simulink model "Simulation_straight_line"  (R2017b)
settings: Solver=ode45  StartTime=0.0  StopTime=inf  RelTol=1e-3  EnableMultiTasking=on
values from neighbouring files (symbols this model uses):
  s = zc-d1    [ArticuledManipulator_Ik.m]
undefined symbols (not defined in the file or in its folder): baza, efector, flansa, robot_nou, RootGround, RootPart, rv
libraries: mblibv1 x31, vrlib x8, simulink x1
settings Model: Creator=elod  LastModifiedBy=Rodrigo Chi
settings DataIOCC: LimitDataPoints=on  SaveFormat=Array  SignalLoggingSaveFormat=ModelDataLogs
settings OptimizationCC: ExpressionDepthLimit=2147483647  LifeSpan=inf
settings DebuggingCC: AlgebraicLoopMsg=none  UnderspecifiedInitializationDetection=Classic  MergeDetectMultiDrivingBlocksExec=none  SolverPrmCheckMsg=warning  FcnCallInpInsideContextMsg=warning  StateNameClashWarn=warning  SFUnexpectedBacktrackingDiag=warning  SFNoUnconditionalDefaultTransitionDiag=warning  SFExecutionAtInitializationDiag=none
settings HardwareCC: ProdBitPerPointer=32  ProdBitPerSizeT=32  ProdBitPerPtrDiffT=32  ProdLargestAtomicFloat=None  ProdIntDivRoundTo=Undefined  ProdEndianess=Unspecified  ProdWordSize=32  ProdHWDeviceType=32-bit Generic
settings ModelReferenceCC: PropagateSignalLabelsOutOfModel=off
settings CodeAppCC: StateflowObjectComments=on
settings GRTTargetCC: TargetLangStandard=C89/C90 (ANSI)  GeneratePreprocessorConditionals=Disable all  CombineOutputUpdateFcns=off  GRTInterface=on
settings ConfigComp: CovMetricSettings=dw  CovHtmlReporting=on  CovSaveCumulativeToWorkspaceVar=on  CovSaveSingleToWorkspaceVar=on  CovExternalEMLEnable=off
settings SimscapeCC: SimscapeNormalizeSystem=off
settings SimMechanicsCC: VisOnUpdateDiagram=on  VisDuringSimulation=on

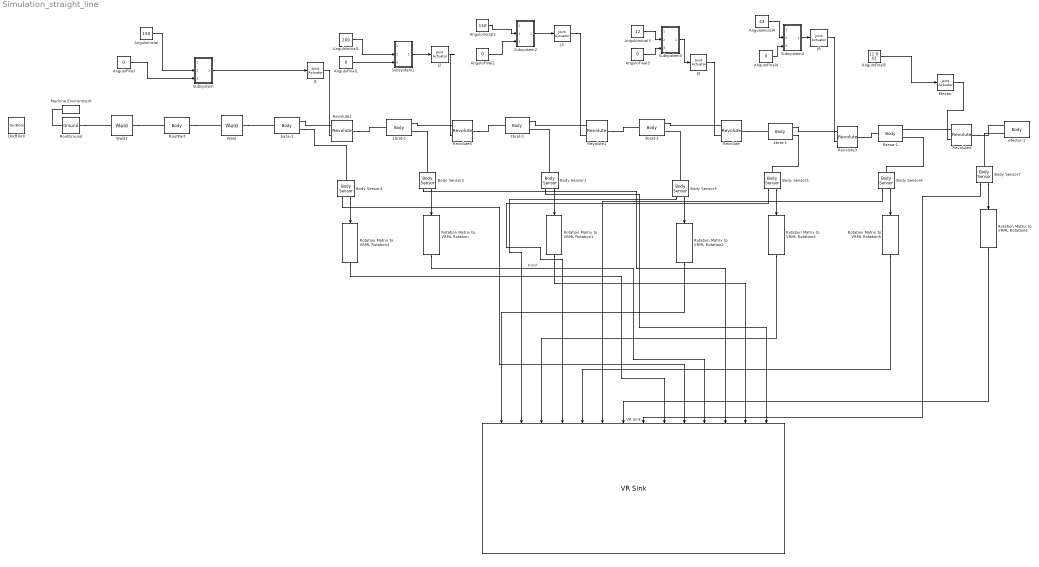
== system Simulation_straight_line ==
  1brat-1 : mblibv1/Bodies/Body  LConnTagsString=CS2  RConnTagsString=CS3|CS4  UpdateFromCAD=on  PMImportedID=1brat-1  DialogClass=MechanicalBodyBlock  Mass=2.25015  MassUnits=kg  InertiaUnits=kg*m^2  Inertia=[0.00885227,-5.51348e-008,-0.000219712;-5.51348e-008,0.00930047,6.21532e-009;-0.000219712,6.21532e-009,0.00500541]  Shape=Cylinder  ShapeDims=[1 1]  ShapeUnits=m  ShapeUse=false  Density=1  DensityUnits=kg/m^3  DensityUse=false  GraphicsMode=GFXFILE  GraphicsFileName=C:\Users\Rodrigo Chi\Desktop\Robot_Melfa\robot_nou - 1brat-1.STL  BodyColorSelMode=COLORPALETTE  BodyColor=[0.65098;0.65098;0.65098]  AttachedToCS=CS1  CG=Right$CG$[0.00726331 0.0794388 -8.78869e-008]$WORLD$WORLD$m$[-1 0 0;0 0 1;0 1 0]$3x3 Transform$rad$WORLD$false$1brat-1::CG(AUTOGEN)  WorkingFrames=Right$CS1$[0 -0.00299998 0]$WORLD$WORLD$m$[-1 0 0;0 0 1;0 1 0]$3x3 Transform$rad$WORLD$false$1brat-1::CS1(AUTOGEN)#Left$CS2$[-1.38778e-017 2.5e-008 5.8564e-016]$WORLD$WORLD$m$[1 0 0;0 1 0;0 0 1]$3x3 Transform$rad$WORLD$true$1brat-1:-:baza-1::1brat-1(AUTOGEN)#Right$CS3$[0 0.1295 -0.0448145]$WORLD$WORLD$m$[1 0 0;0 1 0;0 0 1]$3x3 Transform$rad$WORLD$true$1brat-1:-:2brat-1::1brat-1(AUTOGEN)#Right$CS4$[0 0 0]$WORLD$WORLD$m$[1 0 0;0 1 0;0 0 1]$3x3 Transform$rad$WORLD$true$none  CGPos=[0.00726331 0.0794388 -8.78869e-008]  CGRot=[-1 0 0;0 0 1;0 1 0]  CS0Pos=[]  CS0Rot=[]  CS1Pos=[0 -0.00299998 0]  CS1Rot=[-1 0 0;0 0 1;0 1 0]  CS2Pos=[-1.38778e-017 2.5e-008 5.8564e-016]  CS2Rot=[1 0 0;0 1 0;0 0 1]  CS3Pos=[0 0.1295 -0.0448145]  CS3Rot=[1 0 0;0 1 0;0 0 1]  CS4Pos=[0 0 0]  CS4Rot=[1 0 0;0 1 0;0 0 1]  CS5Pos=[]  CS5Rot=[]  CS6Pos=[]  CS6Rot=[]  CS7Pos=[]  CS7Rot=[]  CS8Pos=[]  CS8Rot=[]  CS9Pos=[]  CS9Rot=[]  CS10Pos=[]  CS10Rot=[]  CS11Pos=[]  CS11Rot=[]  CS12Pos=[]  CS12Rot=[]  CS13Pos=[]  CS13Rot=[]  CS14Pos=[]  CS14Rot=[]  CS15Pos=[]  CS15Rot=[]  CS16Pos=[]  CS16Rot=[]  CS17Pos=[]  CS17Rot=[]  CS18Pos=[]  CS18Rot=[]  CS19Pos=[]  CS19Rot=[]  CS20Pos=[]  CS20Rot=[]
      settings: SourceProductName=Simscape Multibody  SourceProductBaseCode=MS
  2brat-1 : mblibv1/Bodies/Body  LConnTagsString=CS3  RConnTagsString=CS2|CS4  UpdateFromCAD=on  PMImportedID=2brat-1  DialogClass=MechanicalBodyBlock  Mass=3.62743  MassUnits=kg  InertiaUnits=kg*m^2  Inertia=[0.0393757,-7.68618e-009,0.000126615;-7.68618e-009,0.0293486,-4.48119e-008;0.000126615,-4.48119e-008,0.0153003]  Shape=Cylinder  ShapeDims=[1 1]  ShapeUnits=m  ShapeUse=false  Density=1  DensityUnits=kg/m^3  DensityUse=false  GraphicsMode=GFXFILE  GraphicsFileName=C:\Users\Rodrigo Chi\Desktop\Robot_Melfa\robot_nou - 2brat-1.STL  BodyColorSelMode=COLORPALETTE  BodyColor=[0.65098;0.65098;0.65098]  AttachedToCS=CS1  CG=Right$CG$[-0.000659844 0.24353 1.10558e-006]$WORLD$WORLD$m$[1 0 0;0 0 1;0 -1 0]$3x3 Transform$rad$WORLD$false$2brat-1::CG(AUTOGEN)  WorkingFrames=Right$CS1$[0 0.1295 0]$WORLD$WORLD$m$[1 0 0;0 0 1;0 -1 0]$3x3 Transform$rad$WORLD$false$2brat-1::CS1(AUTOGEN)#Right$CS2$[0 0.3795 0.0880007]$WORLD$WORLD$m$[1 0 0;0 1 0;0 0 1]$3x3 Transform$rad$WORLD$true$2brat-1:-:3brat-1::2brat-1(AUTOGEN)#Left$CS3$[0 0.1295 -0.0448145]$WORLD$WORLD$m$[1 0 0;0 1 0;0 0 1]$3x3 Transform$rad$WORLD$true$1brat-1:-:2brat-1::2brat-1(AUTOGEN)#Right$CS4$[0 0 0]$WORLD$WORLD$m$[1 0 0;0 1 0;0 0 1]$3x3 Transform$rad$WORLD$true$none  CGPos=[-0.000659844 0.24353 1.10558e-006]  CGRot=[1 0 0;0 0 1;0 -1 0]  CS0Pos=[]  CS0Rot=[]  CS1Pos=[0 0.1295 0]  CS1Rot=[1 0 0;0 0 1;0 -1 0]  CS2Pos=[0 0.3795 0.0880007]  CS2Rot=[1 0 0;0 1 0;0 0 1]  CS3Pos=[0 0.1295 -0.0448145]  CS3Rot=[1 0 0;0 1 0;0 0 1]  CS4Pos=[0 0 0]  CS4Rot=[1 0 0;0 1 0;0 0 1]  CS5Pos=[]  CS5Rot=[]  CS6Pos=[]  CS6Rot=[]  CS7Pos=[]  CS7Rot=[]  CS8Pos=[]  CS8Rot=[]  CS9Pos=[]  CS9Rot=[]  CS10Pos=[]  CS10Rot=[]  CS11Pos=[]  CS11Rot=[]  CS12Pos=[]  CS12Rot=[]  CS13Pos=[]  CS13Rot=[]  CS14Pos=[]  CS14Rot=[]  CS15Pos=[]  CS15Rot=[]  CS16Pos=[]  CS16Rot=[]  CS17Pos=[]  CS17Rot=[]  CS18Pos=[]  CS18Rot=[]  CS19Pos=[]  CS19Rot=[]  CS20Pos=[]  CS20Rot=[]
      settings: SourceProductName=Simscape Multibody  SourceProductBaseCode=MS
  3brat-1 : mblibv1/Bodies/Body  LConnTagsString=CS3  RConnTagsString=CS2|CS4  UpdateFromCAD=on  PMImportedID=3brat-1  DialogClass=MechanicalBodyBlock  Mass=1.71089  MassUnits=kg  InertiaUnits=kg*m^2  Inertia=[0.00842552,-6.36697e-007,1.27806e-006;-6.36697e-007,0.00773782,1.23963e-005;1.27806e-006,1.23963e-005,0.00280267]  Shape=Cylinder  ShapeDims=[1 1]  ShapeUnits=m  ShapeUse=false  Density=1  DensityUnits=kg/m^3  DensityUse=false  GraphicsMode=GFXFILE  GraphicsFileName=C:\Users\Rodrigo Chi\Desktop\Robot_Melfa\robot_nou - 3brat-1.STL  BodyColorSelMode=COLORPALETTE  BodyColor=[0.65098;0.65098;0.65098]  AttachedToCS=CS1  CG=Right$CG$[7.52531e-006 0.448063 0.00032452]$WORLD$WORLD$m$[1 0 0;0 0 1;0 -1 0]$3x3 Transform$rad$WORLD$false$3brat-1::CG(AUTOGEN)  WorkingFrames=Right$CS1$[0 0.3795 0]$WORLD$WORLD$m$[1 0 0;0 0 1;0 -1 0]$3x3 Transform$rad$WORLD$false$3brat-1::CS1(AUTOGEN)#Right$CS2$[-0.000180127 0.5395 -0.0224506]$WORLD$WORLD$m$[1 0 0;0 1 0;0 0 1]$3x3 Transform$rad$WORLD$true$3brat-1:-:4brat-1::3brat-1(AUTOGEN)#Left$CS3$[0 0.3795 0.0880007]$WORLD$WORLD$m$[1 0 0;0 1 0;0 0 1]$3x3 Transform$rad$WORLD$true$2brat-1:-:3brat-1::3brat-1(AUTOGEN)#Right$CS4$[0 0 0]$WORLD$WORLD$m$[1 0 0;0 1 0;0 0 1]$3x3 Transform$rad$WORLD$true$none  CGPos=[7.52531e-006 0.448063 0.00032452]  CGRot=[1 0 0;0 0 1;0 -1 0]  CS0Pos=[]  CS0Rot=[]  CS1Pos=[0 0.3795 0]  CS1Rot=[1 0 0;0 0 1;0 -1 0]  CS2Pos=[-0.000180127 0.5395 -0.0224506]  CS2Rot=[1 0 0;0 1 0;0 0 1]  CS3Pos=[0 0.3795 0.0880007]  CS3Rot=[1 0 0;0 1 0;0 0 1]  CS4Pos=[0 0 0]  CS4Rot=[1 0 0;0 1 0;0 0 1]  CS5Pos=[]  CS5Rot=[]  CS6Pos=[]  CS6Rot=[]  CS7Pos=[]  CS7Rot=[]  CS8Pos=[]  CS8Rot=[]  CS9Pos=[]  CS9Rot=[]  CS10Pos=[]  CS10Rot=[]  CS11Pos=[]  CS11Rot=[]  CS12Pos=[]  CS12Rot=[]  CS13Pos=[]  CS13Rot=[]  CS14Pos=[]  CS14Rot=[]  CS15Pos=[]  CS15Rot=[]  CS16Pos=[]  CS16Rot=[]  CS17Pos=[]  CS17Rot=[]  CS18Pos=[]  CS18Rot=[]  CS19Pos=[]  CS19Rot=[]  CS20Pos=[]  CS20Rot=[]
      settings: SourceProductName=Simscape Multibody  SourceProductBaseCode=MS
  4brat-1 : mblibv1/Bodies/Body  LConnTagsString=CS2  RConnTagsString=CS3|CS4  UpdateFromCAD=on  PMImportedID=4brat-1  DialogClass=MechanicalBodyBlock  Mass=0.330921  MassUnits=kg  InertiaUnits=kg*m^2  Inertia=[0.000305863,9.08861e-011,-3.82551e-010;9.08861e-011,0.000416962,-1.09526e-009;-3.82551e-010,-1.09526e-009,0.000217954]  Shape=Cylinder  ShapeDims=[1 1]  ShapeUnits=m  ShapeUse=false  Density=1  DensityUnits=kg/m^3  DensityUse=false  GraphicsMode=GFXFILE  GraphicsFileName=C:\Users\Rodrigo Chi\Desktop\Robot_Melfa\robot_nou - 4brat-1.STL  BodyColorSelMode=COLORPALETTE  BodyColor=[0.65098;0.65098;0.65098]  AttachedToCS=CS1  CG=Right$CG$[-0.000180145 0.534322 2.80673e-008]$WORLD$WORLD$m$[1 0 0;0 0 1;0 -1 0]$3x3 Transform$rad$WORLD$false$4brat-1::CG(AUTOGEN)  WorkingFrames=Right$CS1$[-0.000180127 0.5395 0]$WORLD$WORLD$m$[1 0 0;0 0 1;0 -1 0]$3x3 Transform$rad$WORLD$false$4brat-1::CS1(AUTOGEN)#Left$CS2$[-0.000180127 0.5395 -0.0224506]$WORLD$WORLD$m$[1 0 0;0 1 0;0 0 1]$3x3 Transform$rad$WORLD$true$3brat-1:-:4brat-1::4brat-1(AUTOGEN)#Right$CS3$[-0.000180127 0.5855 0]$WORLD$WORLD$m$[1 0 0;0 1 0;0 0 1]$3x3 Transform$rad$WORLD$true$4brat-1:-:flansa-1::4brat-1(AUTOGEN)#Right$CS4$[0 0 0]$WORLD$WORLD$m$[1 0 0;0 1 0;0 0 1]$3x3 Transform$rad$WORLD$true$none  CGPos=[-0.000180145 0.534322 2.80673e-008]  CGRot=[1 0 0;0 0 1;0 -1 0]  CS0Pos=[]  CS0Rot=[]  CS1Pos=[-0.000180127 0.5395 0]  CS1Rot=[1 0 0;0 0 1;0 -1 0]  CS2Pos=[-0.000180127 0.5395 -0.0224506]  CS2Rot=[1 0 0;0 1 0;0 0 1]  CS3Pos=[-0.000180127 0.5855 0]  CS3Rot=[1 0 0;0 1 0;0 0 1]  CS4Pos=[0 0 0]  CS4Rot=[1 0 0;0 1 0;0 0 1]  CS5Pos=[]  CS5Rot=[]  CS6Pos=[]  CS6Rot=[]  CS7Pos=[]  CS7Rot=[]  CS8Pos=[]  CS8Rot=[]  CS9Pos=[]  CS9Rot=[]  CS10Pos=[]  CS10Rot=[]  CS11Pos=[]  CS11Rot=[]  CS12Pos=[]  CS12Rot=[]  CS13Pos=[]  CS13Rot=[]  CS14Pos=[]  CS14Rot=[]  CS15Pos=[]  CS15Rot=[]  CS16Pos=[]  CS16Rot=[]  CS17Pos=[]  CS17Rot=[]  CS18Pos=[]  CS18Rot=[]  CS19Pos=[]  CS19Rot=[]  CS20Pos=[]  CS20Rot=[]
      settings: SourceProductName=Simscape Multibody  SourceProductBaseCode=MS
  AnguloFinal{,1..4} (5 alike) : Constant  Value=0
  AnguloFinal5 : Constant  Value=[1 0 0]
  AnguloInicial : Constant  Value=150
  AnguloInicial1 : Constant  Value=200
  AnguloInicial2 : Constant  Value=150
  AnguloInicial3 : Constant  Value=12
  AnguloInicial4 : Constant  Value=44
  Body Sensor{1..7} (7 alike) : mblibv1/Sensors &  Actuators/Body Sensor  UpdateFromCAD=off  PhysicalDomain=Mechanical  PortType=blob  Muxed=off  Pose=on  Angle=on  AngleUnits=deg  ArcVelocity=off  ArcVelocityUnits=deg/s  ArcAcceleration=off  ArcAccelerationUnits=deg/s^2  CoordPosition=on  CoordPositionUnits=m  Velocity=off  VelocityUnits=m/s  Acceleration=off  AccelerationUnits=m/s^2  Quaternion=on  QuaternionDT=off  QuaternionDDT=off  QuaternionUnits=off  OutputVector=[1]  ActiveIO=on  Width=12  DialogClass=MechanicalSensorBlock  ReferenceFrame=Absolute (World)
      settings: SourceProductName=Simscape Multibody  SourceProductBaseCode=MS
  DocBlock : simulink/Model-Wide Utilities/DocBlock  DocumentType=Text
      content=|
      | Type your documentation here
      | el robot funcioa por bloques y los ejes de rotacion estan unidos
      | a actuadores que a su vez reciben 3 constantes ed las cuales
      | 1 se puede cambiar usando el slider
      |
      | cada eje(revolute) esta basado en l eje del robot
      | hay algunos que solo giran en x y otros en y etc
      | para la manipulacion se usa el slider gain con un rango de -180
      | a 180
      |
      | los join actuator se deben cambiar de "generalized forces" a
      | "motion" para poder ser manipulados
  Efector : mblibv1/Sensors &  Actuators/Joint Actuator  UpdateFromCAD=off  PhysicalDomain=Mechanical  PortType=blob  ActuationStyle=Motion  AngleUnits=deg  ArcVelocityUnits=deg/s  ArcAccelerationUnits=deg/s^2  CoordPositionUnits=m  VelocityUnits=m/s  AccelerationUnits=m/s^2  ForceUnits=N  TorqueUnits=N*m  ActiveIO=on  Width=3  DialogClass=MechanicalActuatorBlock  Primitive=R1  ReferenceFrame=Absolute (World)
      settings: SourceProductName=Simscape Multibody  SourceProductBaseCode=MS
  J{1..3,5..6} (5 alike) : mblibv1/Sensors &  Actuators/Joint Actuator  UpdateFromCAD=off  PhysicalDomain=Mechanical  PortType=blob  ActuationStyle=Motion  AngleUnits=deg  ArcVelocityUnits=deg/s  ArcAccelerationUnits=deg/s^2  CoordPositionUnits=m  VelocityUnits=m/s  AccelerationUnits=m/s^2  ForceUnits=N  TorqueUnits=N*m  ActiveIO=on  Width=3  DialogClass=MechanicalActuatorBlock  Primitive=R1  ReferenceFrame=Absolute (World)
      settings: SourceProductName=Simscape Multibody  SourceProductBaseCode=MS
  Machine Environment : mblibv1/Bodies/Machine Environment  PortType=env  PhysicalDomain=Mechanical  DialogTemplateClass=MECH.MachineEnvironment  SyncWhenCopied=off  Gravity=[0 -9.81 0]  GravityUnits=m/s^2  GravityAsSignal=off  Dimensionality=Auto-detect  AnalysisType=Forward dynamics  LinearAssemblyTolerance=1e-3  LinearAssemblyToleranceUnits=m  AngularAssemblyTolerance=1e-3  AngularAssemblyToleranceUnits=rad  ConstraintSolverType=Stabilizing  ConstraintRelTolerance=1e-4  ConstraintAbsTolerance=1e-4  UseRobustSingularityHandling=off  RedundancyAnalysisToleranceType=Automatically select tolerance  RedundancyAnalysisTolerance=1e-14  StatePerturbationType=Fixed  PerturbationSize=1e-5  VisualizeMachine=on  BodyVisualizationType=Use model default body geometries  BodyColorSelMode=Use model default  DefaultBodyColor=[1 0 0]
      settings: SourceProductName=Simscape Multibody  SourceProductBaseCode=MS
  Revolute : mblibv1/Joints/Revolute  LConnTagsString=__newl0|SA1  RConnTagsString=__newr0  UpdateFromCAD=on  PMImportedID=3brat-1:-:4brat-1  NumSAPorts=1  CutJoint=off  MarkAsCut=off  Primitives=prismatic  PrimitiveProps=R1$World$[0,0,-1]$revolute  DialogClass=JointBlock  R1Axis=[0,0,-1]
      settings: SourceProductName=Simscape Multibody  SourceProductBaseCode=MS
  Revolute1 : mblibv1/Joints/Revolute  LConnTagsString=__newl0|SA1  RConnTagsString=__newr0  UpdateFromCAD=on  PMImportedID=2brat-1:-:3brat-1  NumSAPorts=1  CutJoint=off  MarkAsCut=off  Primitives=prismatic  PrimitiveProps=R1$World$[0,0,-1]$revolute  DialogClass=JointBlock  R1Axis=[0,0,-1]
      settings: SourceProductName=Simscape Multibody  SourceProductBaseCode=MS
  Revolute2 : mblibv1/Joints/Revolute  LConnTagsString=__newl0|SA1  RConnTagsString=__newr0  UpdateFromCAD=on  PMImportedID=1brat-1:-:baza-1  NumSAPorts=1  CutJoint=off  MarkAsCut=off  Primitives=prismatic  PrimitiveProps=R1$World$[0,1,0]$revolute  DialogClass=JointBlock  R1Axis=[0,1,0]
      settings: SourceProductName=Simscape Multibody  SourceProductBaseCode=MS
  Revolute3 : mblibv1/Joints/Revolute  LConnTagsString=__newl0|SA1  RConnTagsString=__newr0  UpdateFromCAD=on  PMImportedID=4brat-1:-:flansa-1  NumSAPorts=1  CutJoint=off  MarkAsCut=off  Primitives=prismatic  PrimitiveProps=R1$World$[0,1,0]$revolute  DialogClass=JointBlock  R1Axis=[0,1,0]
      settings: SourceProductName=Simscape Multibody  SourceProductBaseCode=MS
  Revolute4 : mblibv1/Joints/Revolute  LConnTagsString=__newl0|SA1  RConnTagsString=__newr0  UpdateFromCAD=on  PMImportedID=efector-1:-:flansa-1  NumSAPorts=1  CutJoint=off  MarkAsCut=off  Primitives=prismatic  PrimitiveProps=R1$World$[0,1,0]$revolute  DialogClass=JointBlock  R1Axis=[0,1,0]
      settings: SourceProductName=Simscape Multibody  SourceProductBaseCode=MS
  Revolute5 : mblibv1/Joints/Revolute  LConnTagsString=__newl0|SA1  RConnTagsString=__newr0  UpdateFromCAD=on  PMImportedID=1brat-1:-:2brat-1  NumSAPorts=1  CutJoint=off  MarkAsCut=off  Primitives=prismatic  PrimitiveProps=R1$World$[0,0,1]$revolute  DialogClass=JointBlock  R1Axis=[0,0,1]
      settings: SourceProductName=Simscape Multibody  SourceProductBaseCode=MS
  RootGround : mblibv1/Bodies/Ground  UpdateFromCAD=on  PMImportedID=RootGround  LeftPortType=env  RightPortType=workingframe  PhysicalDomain=Mechanical  DialogClass=GroundBlock  CoordPosition=[0.0162361,0.125438,4.43298e-005]  CoordPositionUnits=m  StateVectorMgrId=3  MachineId=[4 0]  ShowEnvPort=on  ParameterChecksum=[727912128, 70383034, 523039224, 3416024631]  TopologyChecksum=[549250593, 3930916714, 1254666677, 4177042960]
      settings: SourceProductName=Simscape Multibody  SourceProductBaseCode=MS
  RootPart : mblibv1/Bodies/Body  LConnTagsString=CS3  RConnTagsString=CS2  UpdateFromCAD=on  PMImportedID=robot_nou/RootPart  DialogClass=MechanicalBodyBlock  Mass=0  MassUnits=kg  InertiaUnits=kg*m^2  Inertia=[0,0,0;0,0,0;0,0,0]  Shape=Cylinder  ShapeDims=[1 1]  ShapeUnits=m  ShapeUse=false  Density=1  DensityUnits=kg/m^3  DensityUse=false  GraphicsMode=GFXFILE  GraphicsFileName=C:\Users\Rodrigo Chi\Desktop\Robot Físico Geo\Robotsimulado\robot_nou - baza-1.STL  BodyColorSelMode=COLORPALETTE  BodyColor=[0.501961;0.501961;0.501961]  AttachedToCS=CS1  CG=Right$CG$[0.0162361 0.125438 4.43298e-005]$WORLD$WORLD$m$[1 0 0;0 1 0;0 0 1]$3x3 Transform$rad$WORLD$false$robot_nou/RootPart::CG(AUTOGEN)  WorkingFrames=Right$CS1$[0 0 0]$WORLD$WORLD$m$[1 0 0;0 1 0;0 0 1]$3x3 Transform$rad$WORLD$false$robot_nou/RootPart::CS1(AUTOGEN)#Right$CS2$[0.0387863 -0.0914613 7.26852e-006]$WORLD$WORLD$m$[1 0 0;0 1 0;0 0 1]$3x3 Transform$rad$WORLD$true$baza-1:-:robot_nou/RootPart::robot_nou/RootPart(AUTOGEN)#Left$CS3$[0.0162361 0.125438 4.43298e-005]$WORLD$WORLD$m$[1 0 0;0 1 0;0 0 1]$3x3 Transform$rad$WORLD$true$RootGround:-:robot_nou/RootPart::robot_nou/RootPart(AUTOGEN)  CGPos=[0.0162361 0.125438 4.43298e-005]  CGRot=[1 0 0;0 1 0;0 0 1]  CS0Pos=[]  CS0Rot=[]  CS1Pos=[0 0 0]  CS1Rot=[1 0 0;0 1 0;0 0 1]  CS2Pos=[0.0387863 -0.0914613 7.26852e-006]  CS2Rot=[1 0 0;0 1 0;0 0 1]  CS3Pos=[0.0162361 0.125438 4.43298e-005]  CS3Rot=[1 0 0;0 1 0;0 0 1]  CS4Pos=[]  CS4Rot=[]  CS5Pos=[]  CS5Rot=[]  CS6Pos=[]  CS6Rot=[]  CS7Pos=[]  CS7Rot=[]  CS8Pos=[]  CS8Rot=[]  CS9Pos=[]  CS9Rot=[]  CS10Pos=[]  CS10Rot=[]  CS11Pos=[]  CS11Rot=[]  CS12Pos=[]  CS12Rot=[]  CS13Pos=[]  CS13Rot=[]  CS14Pos=[]  CS14Rot=[]  CS15Pos=[]  CS15Rot=[]  CS16Pos=[]  CS16Rot=[]  CS17Pos=[]  CS17Rot=[]  CS18Pos=[]  CS18Rot=[]  CS19Pos=[]  CS19Rot=[]  CS20Pos=[]  CS20Rot=[]
      settings: SourceProductName=Simscape Multibody  SourceProductBaseCode=MS
  Rotation Matrix to VRML Rotation{,1..6} (7 alike) : vrlib/Utilities/Rotation Matrix to VRML Rotation  maxzero=1e-12
      settings: SourceProductName=Simulink 3D Animation  SourceProductBaseCode=VR
  Subsystem : Subsystem
  Subsystem1 : Subsystem
  Subsystem2 : Subsystem
  Subsystem3 : Subsystem
  Subsystem4 : Subsystem
  VR Sink : vrlib/VR Sink  InstantiateOnLoad=on  SampleTime=0.1  ViewEnable=on  RemoteChange=off  RemoteView=off  FieldsWritten=b3.rotation.4.1.1.double#b3.translation.3.1.1.double#b4.rotation.4.1.1.double#b4.translation.3.1.1.double#f.rotation.4.1.1.double#f.translation.3.1.1.double#e.rotation.4.1.1.double#e.translation.3.1.1.double#bb.rotation.4.1.1.double#bb.translation.3.1.1.double#b1.rotation.4.1.1.double#b1.translation.3.1.1.double#b2.rotation.4.1.1.double#b2.translation.3.1.1.double  WorldFileName=robot_Rva2j.wrl  WorldDescription=rv-2aj  AutoView=off  VideoDimensions=[]  AllowVariableSize=off
      settings: SourceProductBaseCode=VR
  Weld : mblibv1/Joints/Weld  LConnTagsString=__newl0  RConnTagsString=__newr0  UpdateFromCAD=on  PMImportedID=baza-1:-:robot_nou/RootPart  NumSAPorts=0  CutJoint=off  MarkAsCut=off  Primitives=weld  PrimitiveProps=W$WORLD$[0.57735,0.57735,0.57735]$weld  DialogClass=JointBlock  WAxis=[0.57735,0.57735,0.57735]
      settings: SourceProductName=Simscape Multibody  SourceProductBaseCode=MS
  Weld1 : mblibv1/Joints/Weld  LConnTagsString=__newl0  RConnTagsString=__newr0  UpdateFromCAD=on  PMImportedID=RootGround:-:robot_nou/RootPart  NumSAPorts=0  CutJoint=off  MarkAsCut=off  Primitives=weld  PrimitiveProps=W$WORLD$[0.57735,0.57735,0.57735]$weld  DialogClass=JointBlock  WAxis=[0.57735,0.57735,0.57735]
      settings: SourceProductName=Simscape Multibody  SourceProductBaseCode=MS
  baza-1 : mblibv1/Bodies/Body  LConnTagsString=CS2  RConnTagsString=CS3|CS4  UpdateFromCAD=on  PMImportedID=baza-1  DialogClass=MechanicalBodyBlock  Mass=5.28442  MassUnits=kg  InertiaUnits=kg*m^2  Inertia=[0.0219514,4.64467e-006,-0.00187329;4.64467e-006,0.0327268,7.62797e-007;-0.00187329,7.62797e-007,0.0305246]  Shape=Cylinder  ShapeDims=[1 1]  ShapeUnits=m  ShapeUse=false  Density=1  DensityUnits=kg/m^3  DensityUse=false  GraphicsMode=GFXFILE  GraphicsFileName=C:\Users\Rodrigo Chi\Desktop\Robot_Melfa\robot_nou - baza-1.STL  BodyColorSelMode=COLORPALETTE  BodyColor=[0.65098;0.65098;0.65098]  AttachedToCS=CS1  CG=Right$CG$[0.0387863 -0.0914613 7.26852e-006]$WORLD$WORLD$m$[-1 0 0;0 0 1;0 1 0]$3x3 Transform$rad$WORLD$false$baza-1::CG(AUTOGEN)  WorkingFrames=Right$CS1$[0 -0.168 0]$WORLD$WORLD$m$[-1 0 0;0 0 1;0 1 0]$3x3 Transform$rad$WORLD$false$baza-1::CS1(AUTOGEN)#Left$CS2$[0.0387863 -0.0914613 7.26852e-006]$WORLD$WORLD$m$[1 0 0;0 1 0;0 0 1]$3x3 Transform$rad$WORLD$true$baza-1:-:robot_nou/RootPart::baza-1(AUTOGEN)#Right$CS3$[-1.38778e-017 2.5e-008 5.8564e-016]$WORLD$WORLD$m$[1 0 0;0 1 0;0 0 1]$3x3 Transform$rad$WORLD$true$1brat-1:-:baza-1::baza-1(AUTOGEN)#Right$CS4$[0 0 0]$WORLD$WORLD$m$[1 0 0;0 1 0;0 0 1]$3x3 Transform$rad$WORLD$true$none  CGPos=[0.0387863 -0.0914613 7.26852e-006]  CGRot=[-1 0 0;0 0 1;0 1 0]  CS0Pos=[]  CS0Rot=[]  CS1Pos=[0 -0.168 0]  CS1Rot=[-1 0 0;0 0 1;0 1 0]  CS2Pos=[0.0387863 -0.0914613 7.26852e-006]  CS2Rot=[1 0 0;0 1 0;0 0 1]  CS3Pos=[-1.38778e-017 2.5e-008 5.8564e-016]  CS3Rot=[1 0 0;0 1 0;0 0 1]  CS4Pos=[0 0 0]  CS4Rot=[1 0 0;0 1 0;0 0 1]  CS5Pos=[]  CS5Rot=[]  CS6Pos=[]  CS6Rot=[]  CS7Pos=[]  CS7Rot=[]  CS8Pos=[]  CS8Rot=[]  CS9Pos=[]  CS9Rot=[]  CS10Pos=[]  CS10Rot=[]  CS11Pos=[]  CS11Rot=[]  CS12Pos=[]  CS12Rot=[]  CS13Pos=[]  CS13Rot=[]  CS14Pos=[]  CS14Rot=[]  CS15Pos=[]  CS15Rot=[]  CS16Pos=[]  CS16Rot=[]  CS17Pos=[]  CS17Rot=[]  CS18Pos=[]  CS18Rot=[]  CS19Pos=[]  CS19Rot=[]  CS20Pos=[]  CS20Rot=[]
      settings: SourceProductName=Simscape Multibody  SourceProductBaseCode=MS
  efector-1 : mblibv1/Bodies/Body  LConnTagsString=CS2|CS3  UpdateFromCAD=on  PMImportedID=efector-1  DialogClass=MechanicalBodyBlock  Mass=0.170431  MassUnits=kg  InertiaUnits=kg*m^2  Inertia=[0.000106215,-1.25677e-006,2.43146e-015;-1.25677e-006,0.00010751,1.48259e-015;2.43146e-015,1.48259e-015,0.000156336]  Shape=Cylinder  ShapeDims=[1 1]  ShapeUnits=m  ShapeUse=false  Density=1  DensityUnits=kg/m^3  DensityUse=false  GraphicsMode=GFXFILE  GraphicsFileName=C:\Users\Rodrigo Chi\Desktop\Robot_Melfa\robot_nou - efector-1.STL  BodyColorSelMode=COLORPALETTE  BodyColor=[0.65098;0.65098;0.65098]  AttachedToCS=CS1  CG=Right$CG$[-0.000180127 0.62715 0]$WORLD$WORLD$m$[1 0 0;0 0 1;0 -1 0]$3x3 Transform$rad$WORLD$false$efector-1::CG(AUTOGEN)  WorkingFrames=Right$CS1$[-0.000180127 0.6048 0]$WORLD$WORLD$m$[1 0 0;0 0 1;0 -1 0]$3x3 Transform$rad$WORLD$false$efector-1::CS1(AUTOGEN)#Left$CS2$[-0.000180127 0.6048 0]$WORLD$WORLD$m$[1 0 0;0 1 0;0 0 1]$3x3 Transform$rad$WORLD$true$efector-1:-:flansa-1::efector-1(AUTOGEN)#Left$CS3$[0 0 0]$WORLD$WORLD$m$[1 0 0;0 1 0;0 0 1]$3x3 Transform$rad$WORLD$true$none  CGPos=[-0.000180127 0.62715 0]  CGRot=[1 0 0;0 0 1;0 -1 0]  CS0Pos=[]  CS0Rot=[]  CS1Pos=[-0.000180127 0.6048 0]  CS1Rot=[1 0 0;0 0 1;0 -1 0]  CS2Pos=[-0.000180127 0.6048 0]  CS2Rot=[1 0 0;0 1 0;0 0 1]  CS3Pos=[0 0 0]  CS3Rot=[1 0 0;0 1 0;0 0 1]  CS4Pos=[]  CS4Rot=[]  CS5Pos=[]  CS5Rot=[]  CS6Pos=[]  CS6Rot=[]  CS7Pos=[]  CS7Rot=[]  CS8Pos=[]  CS8Rot=[]  CS9Pos=[]  CS9Rot=[]  CS10Pos=[]  CS10Rot=[]  CS11Pos=[]  CS11Rot=[]  CS12Pos=[]  CS12Rot=[]  CS13Pos=[]  CS13Rot=[]  CS14Pos=[]  CS14Rot=[]  CS15Pos=[]  CS15Rot=[]  CS16Pos=[]  CS16Rot=[]  CS17Pos=[]  CS17Rot=[]  CS18Pos=[]  CS18Rot=[]  CS19Pos=[]  CS19Rot=[]  CS20Pos=[]  CS20Rot=[]
      settings: SourceProductName=Simscape Multibody  SourceProductBaseCode=MS
  flansa-1 : mblibv1/Bodies/Body  LConnTagsString=CS2  RConnTagsString=CS3|CS4  UpdateFromCAD=on  PMImportedID=flansa-1  DialogClass=MechanicalBodyBlock  Mass=0.103138  MassUnits=kg  InertiaUnits=kg*m^2  Inertia=[4.34781e-005,0,-2.81871e-008;0,4.34391e-005,0;-2.81871e-008,0,7.89834e-005]  Shape=Cylinder  ShapeDims=[1 1]  ShapeUnits=m  ShapeUse=false  Density=1  DensityUnits=kg/m^3  DensityUse=false  GraphicsMode=GFXFILE  GraphicsFileName=C:\Users\Rodrigo Chi\Desktop\Robot_Melfa\robot_nou - flansa-1.STL  BodyColorSelMode=COLORPALETTE  BodyColor=[0;1;1]  AttachedToCS=CS1  CG=Right$CG$[-0.00015614 0.595907 0]$WORLD$WORLD$m$[1 0 0;0 0 1;0 -1 0]$3x3 Transform$rad$WORLD$false$flansa-1::CG(AUTOGEN)  WorkingFrames=Right$CS1$[-0.000180127 0.6113 0]$WORLD$WORLD$m$[1 0 0;0 0 1;0 -1 0]$3x3 Transform$rad$WORLD$false$flansa-1::CS1(AUTOGEN)#Left$CS2$[-0.000180127 0.5855 0]$WORLD$WORLD$m$[1 0 0;0 1 0;0 0 1]$3x3 Transform$rad$WORLD$true$4brat-1:-:flansa-1::flansa-1(AUTOGEN)#Right$CS3$[-0.000180127 0.6048 0]$WORLD$WORLD$m$[1 0 0;0 1 0;0 0 1]$3x3 Transform$rad$WORLD$true$efector-1:-:flansa-1::flansa-1(AUTOGEN)#Right$CS4$[0 0 0]$WORLD$WORLD$m$[1 0 0;0 1 0;0 0 1]$3x3 Transform$rad$WORLD$true$none  CGPos=[-0.00015614 0.595907 0]  CGRot=[1 0 0;0 0 1;0 -1 0]  CS0Pos=[]  CS0Rot=[]  CS1Pos=[-0.000180127 0.6113 0]  CS1Rot=[1 0 0;0 0 1;0 -1 0]  CS2Pos=[-0.000180127 0.5855 0]  CS2Rot=[1 0 0;0 1 0;0 0 1]  CS3Pos=[-0.000180127 0.6048 0]  CS3Rot=[1 0 0;0 1 0;0 0 1]  CS4Pos=[0 0 0]  CS4Rot=[1 0 0;0 1 0;0 0 1]  CS5Pos=[]  CS5Rot=[]  CS6Pos=[]  CS6Rot=[]  CS7Pos=[]  CS7Rot=[]  CS8Pos=[]  CS8Rot=[]  CS9Pos=[]  CS9Rot=[]  CS10Pos=[]  CS10Rot=[]  CS11Pos=[]  CS11Rot=[]  CS12Pos=[]  CS12Rot=[]  CS13Pos=[]  CS13Rot=[]  CS14Pos=[]  CS14Rot=[]  CS15Pos=[]  CS15Rot=[]  CS16Pos=[]  CS16Rot=[]  CS17Pos=[]  CS17Rot=[]  CS18Pos=[]  CS18Rot=[]  CS19Pos=[]  CS19Rot=[]  CS20Pos=[]  CS20Rot=[]
      settings: SourceProductName=Simscape Multibody  SourceProductBaseCode=MS
  wires:
  Body Sensor2/2 -> Rotation Matrix to VRML Rotation/1
  Body Sensor1/2 -> Rotation Matrix to VRML Rotation1/1
  Body Sensor3/2 -> Rotation Matrix to VRML Rotation2/1
  Rotation Matrix to VRML Rotation2/1 -> VR Sink/1
  Body Sensor3/1 -> VR Sink/2
  Rotation Matrix to VRML Rotation1/1 -> VR Sink/13
  Body Sensor1/1 -> VR Sink/14
  Rotation Matrix to VRML Rotation/1 -> VR Sink/11  "Dddsf"
  Body Sensor2/1 -> VR Sink/12
  Body Sensor4/2 -> Rotation Matrix to VRML Rotation3/1
  Rotation Matrix to VRML Rotation3/1 -> VR Sink/9
  Body Sensor4/1 -> VR Sink/10
  Body Sensor5/2 -> Rotation Matrix to VRML Rotation4/1
  Rotation Matrix to VRML Rotation4/1 -> VR Sink/3
  Body Sensor5/1 -> VR Sink/4
  Body Sensor6/2 -> Rotation Matrix to VRML Rotation5/1
  Rotation Matrix to VRML Rotation5/1 -> VR Sink/5
  Body Sensor6/1 -> VR Sink/6
  Body Sensor7/2 -> Rotation Matrix to VRML Rotation6/1
  Rotation Matrix to VRML Rotation6/1 -> VR Sink/7
  Body Sensor7/1 -> VR Sink/8
  AnguloInicial/1 -> Subsystem/2(In2)
  AnguloInicial1/1 -> Subsystem1/2(In2)
  AnguloFinal1/1 -> Subsystem1/3(In3)
  Subsystem1/1(Out1) -> J2/1
  AnguloInicial2/1 -> Subsystem2/2(In2)
  AnguloFinal2/1 -> Subsystem2/3(In3)
  Subsystem2/1(Out1) -> J3/1
  AnguloInicial3/1 -> Subsystem3/2(In2)
  AnguloFinal3/1 -> Subsystem3/3(In3)
  AnguloInicial4/1 -> Subsystem4/2(In2)
  AnguloFinal4/1 -> Subsystem4/3(In3)
  Subsystem4/1(Out1) -> J6/1
  AnguloFinal/1 -> Subsystem/3(In3)
  Subsystem/1(Out1) -> J1/1
  AnguloFinal5/1 -> Efector/1
  Subsystem3/1(Out1) -> J5/1
  connections:
  RootPart/RConn1 -- Weld/LConn1
  Weld/RConn1 -- baza-1/LConn1
  3brat-1/RConn1 -- Revolute/LConn1
  Revolute/RConn1 -- 4brat-1/LConn1
  2brat-1/RConn1 -- Revolute1/LConn1
  Revolute1/RConn1 -- 3brat-1/LConn1
  Revolute2/RConn1 -- 1brat-1/LConn1
  4brat-1/RConn1 -- Revolute3/LConn1
  Revolute3/RConn1 -- flansa-1/LConn1
  flansa-1/RConn1 -- Revolute4/LConn1
  Revolute4/RConn1 -- efector-1/LConn1
  1brat-1/RConn1 -- Revolute5/LConn1
  Revolute5/RConn1 -- 2brat-1/LConn1
  RootGround/RConn1 -- Weld1/LConn1
  Weld1/RConn1 -- RootPart/LConn1
  RootGround/LConn1 -- Machine Environment/RConn1
  baza-1/RConn1 -- Revolute2/LConn1
  1brat-1/RConn2 -- Body Sensor2/LConn1
  Body Sensor1/LConn1 -- 2brat-1/RConn2
  Body Sensor3/LConn1 -- 3brat-1/RConn2
  baza-1/RConn2 -- Body Sensor4/LConn1
  4brat-1/RConn2 -- Body Sensor5/LConn1
  Body Sensor6/LConn1 -- flansa-1/RConn2
  Body Sensor7/LConn1 -- efector-1/LConn2
  Efector/RConn1 -- Revolute4/LConn2
  J5/RConn1 -- Revolute/LConn2
  J6/RConn1 -- Revolute3/LConn2
  J1/RConn1 -- Revolute2/LConn2
  J2/RConn1 -- Revolute5/LConn2
  J3/RConn1 -- Revolute1/LConn2

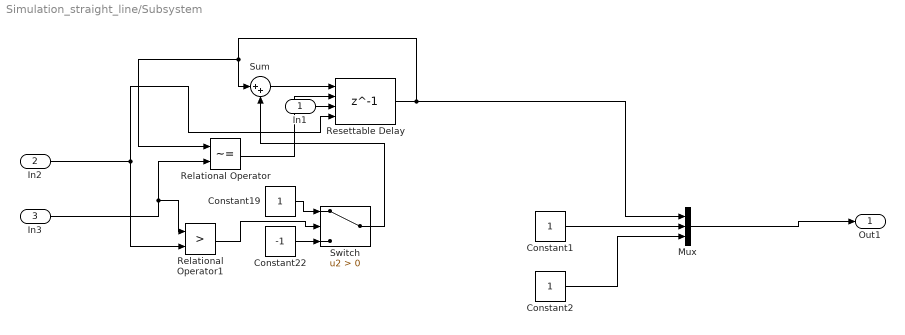
== system Simulation_straight_line/Subsystem ==
  In1 : Inport
  In2 : Inport  Port=2
  In3 : Inport  Port=3
  Constant1 : Constant
  Constant19 : Constant
  Constant2 : Constant
  Constant22 : Constant  Value=-1
  Mux : Mux  Inputs=3
  Relational Operator : RelationalOperator  Operator=~=  OutDataTypeStr=boolean  RndMeth=Simplest
  Relational Operator1 : RelationalOperator  Operator=>  OutDataTypeStr=boolean  RndMeth=Simplest
  Resettable Delay : Delay  DelayLength=1  InitialConditionSource=Input port  ExternalReset=Level  ShowEnablePort=on
      settings: InputPortMap=u0,e6,r5,p4
  Sum : Sum  Inputs=|++
  Switch : Switch  Criteria=u2 > Threshold
  Out1 : Outport
  wires:
  In1/1 -> Resettable Delay/3
  Constant2/1 -> Mux/3
  Constant1/1 -> Mux/2
  Mux/1 -> Out1/1
  Resettable Delay/1 -> Relational Operator/1, Sum/1, Mux/1
  Sum/1 -> Resettable Delay/1
  Relational Operator/1 -> Resettable Delay/2
  Constant22/1 -> Switch/3
  Switch/1 -> Sum/2
  Constant19/1 -> Switch/1
  In2/1 -> Resettable Delay/4, Relational Operator1/2
  In3/1 -> Relational Operator1/1, Relational Operator/2
  Relational Operator1/1 -> Switch/2

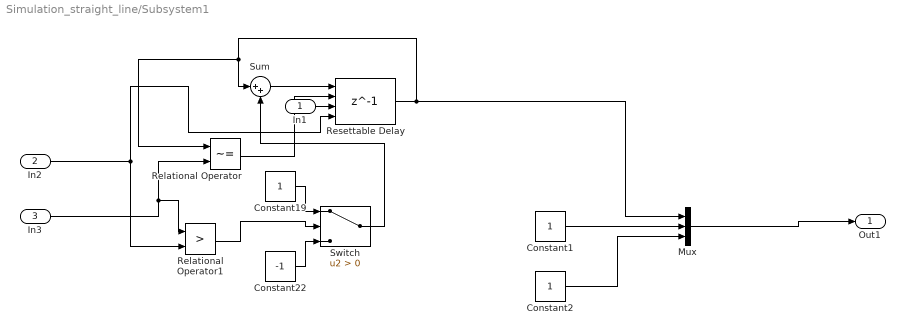
== system Simulation_straight_line/Subsystem1 ==
  In1 : Inport
  In2 : Inport  Port=2
  In3 : Inport  Port=3
  Constant1 : Constant
  Constant19 : Constant
  Constant2 : Constant
  Constant22 : Constant  Value=-1
  Mux : Mux  Inputs=3
  Relational Operator : RelationalOperator  Operator=~=  OutDataTypeStr=boolean  RndMeth=Simplest
  Relational Operator1 : RelationalOperator  Operator=>  OutDataTypeStr=boolean  RndMeth=Simplest
  Resettable Delay : Delay  DelayLength=1  InitialConditionSource=Input port  ExternalReset=Level  ShowEnablePort=on
      settings: InputPortMap=u0,e6,r5,p4
  Sum : Sum  Inputs=|++
  Switch : Switch  Criteria=u2 > Threshold
  Out1 : Outport
  wires:
  In1/1 -> Resettable Delay/3
  Constant2/1 -> Mux/3
  Constant1/1 -> Mux/2
  Mux/1 -> Out1/1
  Resettable Delay/1 -> Relational Operator/1, Sum/1, Mux/1
  Sum/1 -> Resettable Delay/1
  Relational Operator/1 -> Resettable Delay/2
  Constant22/1 -> Switch/3
  Switch/1 -> Sum/2
  Constant19/1 -> Switch/1
  In2/1 -> Resettable Delay/4, Relational Operator1/2
  In3/1 -> Relational Operator1/1, Relational Operator/2
  Relational Operator1/1 -> Switch/2

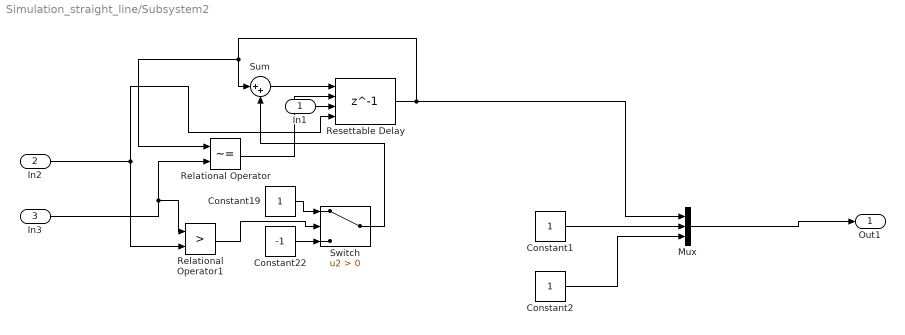
== system Simulation_straight_line/Subsystem2 ==
  In1 : Inport
  In2 : Inport  Port=2
  In3 : Inport  Port=3
  Constant1 : Constant
  Constant19 : Constant
  Constant2 : Constant
  Constant22 : Constant  Value=-1
  Mux : Mux  Inputs=3
  Relational Operator : RelationalOperator  Operator=~=  OutDataTypeStr=boolean  RndMeth=Simplest
  Relational Operator1 : RelationalOperator  Operator=>  OutDataTypeStr=boolean  RndMeth=Simplest
  Resettable Delay : Delay  DelayLength=1  InitialConditionSource=Input port  ExternalReset=Level  ShowEnablePort=on
      settings: InputPortMap=u0,e6,r5,p4
  Sum : Sum  Inputs=|++
  Switch : Switch  Criteria=u2 > Threshold
  Out1 : Outport
  wires:
  In1/1 -> Resettable Delay/3
  Constant2/1 -> Mux/3
  Constant1/1 -> Mux/2
  Mux/1 -> Out1/1
  Resettable Delay/1 -> Relational Operator/1, Sum/1, Mux/1
  Sum/1 -> Resettable Delay/1
  Relational Operator/1 -> Resettable Delay/2
  Constant22/1 -> Switch/3
  Switch/1 -> Sum/2
  Constant19/1 -> Switch/1
  In2/1 -> Resettable Delay/4, Relational Operator1/2
  In3/1 -> Relational Operator1/1, Relational Operator/2
  Relational Operator1/1 -> Switch/2

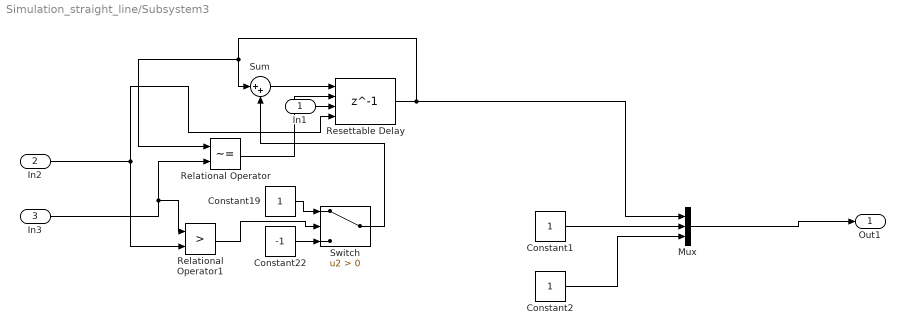
== system Simulation_straight_line/Subsystem3 ==
  In1 : Inport
  In2 : Inport  Port=2
  In3 : Inport  Port=3
  Constant1 : Constant
  Constant19 : Constant
  Constant2 : Constant
  Constant22 : Constant  Value=-1
  Mux : Mux  Inputs=3
  Relational Operator : RelationalOperator  Operator=~=  OutDataTypeStr=boolean  RndMeth=Simplest
  Relational Operator1 : RelationalOperator  Operator=>  OutDataTypeStr=boolean  RndMeth=Simplest
  Resettable Delay : Delay  DelayLength=1  InitialConditionSource=Input port  ExternalReset=Level  ShowEnablePort=on
      settings: InputPortMap=u0,e6,r5,p4
  Sum : Sum  Inputs=|++
  Switch : Switch  Criteria=u2 > Threshold
  Out1 : Outport
  wires:
  In1/1 -> Resettable Delay/3
  Constant2/1 -> Mux/3
  Constant1/1 -> Mux/2
  Mux/1 -> Out1/1
  Resettable Delay/1 -> Relational Operator/1, Sum/1, Mux/1
  Sum/1 -> Resettable Delay/1
  Relational Operator/1 -> Resettable Delay/2
  Constant22/1 -> Switch/3
  Switch/1 -> Sum/2
  Constant19/1 -> Switch/1
  In2/1 -> Resettable Delay/4, Relational Operator1/2
  In3/1 -> Relational Operator1/1, Relational Operator/2
  Relational Operator1/1 -> Switch/2

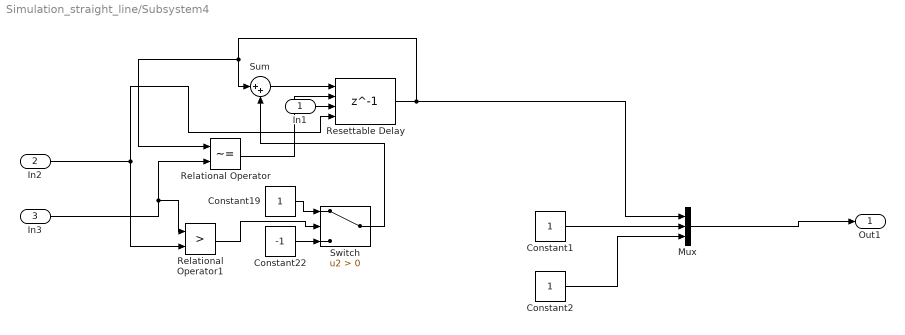
== system Simulation_straight_line/Subsystem4 ==
  In1 : Inport
  In2 : Inport  Port=2
  In3 : Inport  Port=3
  Constant1 : Constant
  Constant19 : Constant
  Constant2 : Constant
  Constant22 : Constant  Value=-1
  Mux : Mux  Inputs=3
  Relational Operator : RelationalOperator  Operator=~=  OutDataTypeStr=boolean  RndMeth=Simplest
  Relational Operator1 : RelationalOperator  Operator=>  OutDataTypeStr=boolean  RndMeth=Simplest
  Resettable Delay : Delay  DelayLength=1  InitialConditionSource=Input port  ExternalReset=Level  ShowEnablePort=on
      settings: InputPortMap=u0,e6,r5,p4
  Sum : Sum  Inputs=|++
  Switch : Switch  Criteria=u2 > Threshold
  Out1 : Outport
  wires:
  In1/1 -> Resettable Delay/3
  Constant2/1 -> Mux/3
  Constant1/1 -> Mux/2
  Mux/1 -> Out1/1
  Resettable Delay/1 -> Relational Operator/1, Sum/1, Mux/1
  Sum/1 -> Resettable Delay/1
  Relational Operator/1 -> Resettable Delay/2
  Constant22/1 -> Switch/3
  Switch/1 -> Sum/2
  Constant19/1 -> Switch/1
  In2/1 -> Resettable Delay/4, Relational Operator1/2
  In3/1 -> Relational Operator1/1, Relational Operator/2
  Relational Operator1/1 -> Switch/2
